simulink model "depth_follower"  (R2019a)
settings: Solver=FixedStepAuto  StartTime=0.0  StopTime=inf  FixedStep=0.1  RelTol=1e-3
model workspace (MAT data in the model file):
  SL_ROS_VariableLengthArrays_MaxSizes.CommonInfo.ArrayTruncateAction = 'EmitWarning'
  SL_ROS_VariableLengthArrays_MaxSizes.MsgTypeMap = containers.Map
  SL_ROS_VariableLengthArrays_MaxSizes.MsgTypeMap.serialization.keys = {'sensor_msgs/Image'}
  SL_ROS_VariableLengthArrays_MaxSizes.MsgTypeMap.serialization.values{1}(1).PropertyName = 'Data'
  SL_ROS_VariableLengthArrays_MaxSizes.MsgTypeMap.serialization.values{1}(1).DataType = 'uint8'
  SL_ROS_VariableLengthArrays_MaxSizes.MsgTypeMap.serialization.values{1}(1).MaxLength = 614400
  SL_ROS_VariableLengthArrays_MaxSizes.MsgTypeMap.serialization.values{1}(2).PropertyName = 'Encoding'
  SL_ROS_VariableLengthArrays_MaxSizes.MsgTypeMap.serialization.values{1}(2).DataType = 'uint8'
  SL_ROS_VariableLengthArrays_MaxSizes.MsgTypeMap.serialization.values{1}(2).MaxLength = 128
  SL_ROS_VariableLengthArrays_MaxSizes.MsgTypeMap.serialization.uniformity = 0
  SL_ROS_VariableLengthArrays_MaxSizes.MsgTypeMap.serialization.keyType = 'char'
  SL_ROS_VariableLengthArrays_MaxSizes.MsgTypeMap.serialization.valueType = 'any'
undefined symbols (not defined in the file): Angular, Linear
libraries: robotlib x5, visionsinks x1
settings Model: EnablePacing=on  Creator=scastro  LastModifiedBy=scastro
settings OptimizationCC: EnhancedBackFolding=on  PassReuseOutputArgsAs=Individual arguments  MaxStackSize=64  OptimizeBlockOrder=speed  DifferentSizesBufferReuse=on  OptimizationCustomize=off
settings DebuggingCC: ParameterTunabilityLossMsg=error
settings HardwareCC: ProdBitPerPointer=32  ProdBitPerSizeT=32  ProdBitPerPtrDiffT=32  ProdLargestAtomicFloat=None  ProdIntDivRoundTo=Undefined  ProdEndianess=Unspecified  ProdWordSize=32  ProdHWDeviceType=Generic->Unspecified (assume 32-bit Generic)
settings RTWCC: SystemTargetFile=ert.tlc  HardwareBoard=Robot Operating System (ROS)  TLCOptions="-aInlineSetEventsForThisBaseRateFcn=TLC_FALSE -aSuppressMultiTaskScheduler=TLC_FALSE  -aRateBasedStepFcn=0"  TemplateMakefile=ert_default_tmf  GenerateReport=on  Toolchain=Catkin  IncludeHyperlinkInReport=on  LaunchReport=on  TargetLang=C++  GenerateTraceInfo=on  GenerateTraceReport=on  GenerateTraceReportSl=on  GenerateTraceReportSf=on  GenerateTraceReportEml=on
settings CodeAppCC: ForceParamTrailComments=on  IgnoreCustomStorageClasses=off  OperatorAnnotations=on  SimulinkDataObjDesc=on  SFDataObjDesc=on  InsertBlockDesc=on
settings ERTTargetCC: SupportVariableSizeSignals=on

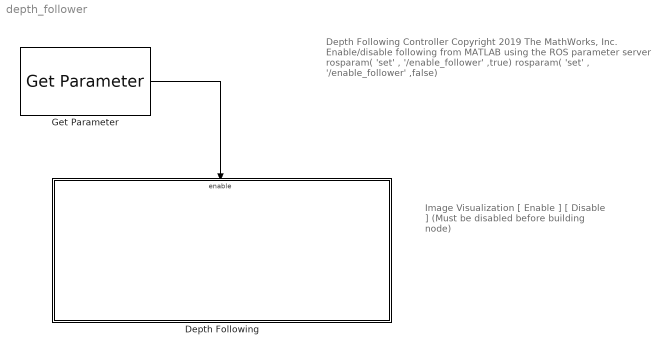
== system depth_follower ==
  note: Depth Following Controller
      | Copyright 2019 The MathWorks, Inc.
      |
      | Enable/disable following from MATLAB
      | using the ROS parameter server
      |
      | rosparam( 'set' , '/enable_follower' ,true)
      | rosparam( 'set' , '/enable_follower' ,false)
  note: Image Visualization
      | [ Enable ] [ Disable ]
      |
      | (Must be disabled before building node)
  Depth Following : Subsystem
  Get Parameter : robotlib/Get Parameter  ParameterSource=Select from ROS network  ParameterName=/enable_follower  ParameterType=boolean  ParameterMaxArrayLength=16  ParameterInitialValue=true  SampleTime=-1  ShowErrorCodeOutput=off  ModelName=depth_follower  BlockId=ParamGet_depth_follower_56
      settings: SourceProductName=Robotics System Toolbox  SourceProductBaseCode=RO
  wires:
  Get Parameter/1 -> Depth Following/Enable

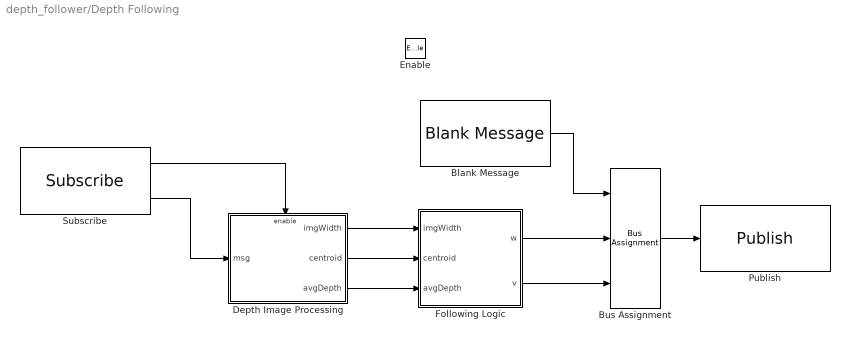
== system depth_follower/Depth Following ==
  Enable : EnablePort
  Blank Message : robotlib/Blank Message  messageClass=Message  entityType=geometry_msgs/Twist  messageType=geometry_msgs/Twist  SampleTime=inf
      settings: SourceProductBaseCode=RO
  Bus Assignment : BusAssignment  AssignedSignals=Angular.Z,Linear.X
  Depth Image Processing : Subsystem
  Following Logic : Subsystem
  Publish : robotlib/Publish  topicSource=Select from ROS network  topic=/mobile_base/commands/velocity  messageType=geometry_msgs/Twist  messageQueueLength=1
      settings: SourceProductBaseCode=RO
  Subscribe : robotlib/Subscribe  topicSource=Select from ROS network  topic=/camera/depth_registered/image_raw  messageType=sensor_msgs/Image  sampleTime=-1  messageQueueLength=1
      settings: SourceProductBaseCode=RO
  wires:
  Blank Message/1 -> Bus Assignment/1
  Depth Image Processing/2(centroid) -> Following Logic/2(centroid)
  Following Logic/1(w) -> Bus Assignment/2
  Following Logic/2(v) -> Bus Assignment/3
  Bus Assignment/1 -> Publish/1
  Depth Image Processing/3(avgDepth) -> Following Logic/3(avgDepth)
  Subscribe/1 -> Depth Image Processing/Enable
  Subscribe/2 -> Depth Image Processing/1(msg)
  Depth Image Processing/1(imgWidth) -> Following Logic/1(imgWidth)

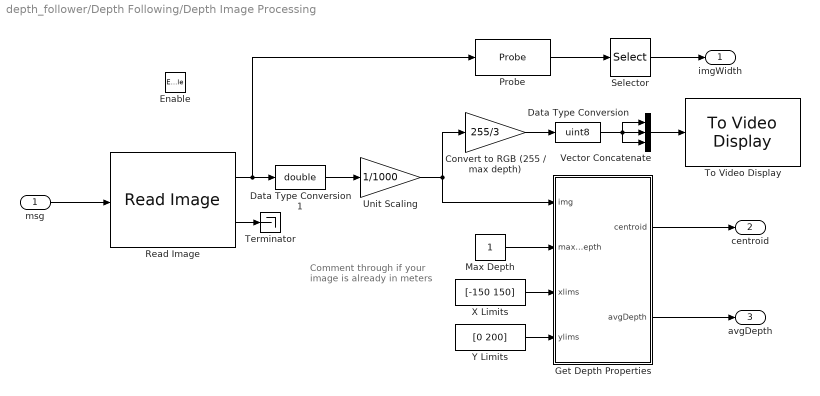
== system depth_follower/Depth Following/Depth Image Processing ==
  note: Comment through if your image is already in meters
  msg : Inport
  Enable : EnablePort
  Convert to RGB (255 / max depth) : Gain  Gain=255/3
  Data Type Conversion : DataTypeConversion  OutDataTypeStr=uint8
  Data Type Conversion1 : DataTypeConversion  OutDataTypeStr=double
  Get Depth Properties : MATLAB Function  TreatAsAtomicUnit=on
  Max Depth : Constant
  Probe : Probe  ProbeWidth=off  ProbeSampleTime=off  ProbeComplexSignal=off  ProbeSignalDimensions=on
  Read Image : robotlib/Read Image  MaximumImageSize=[480, 640]  ImageEncoding=16uc1  ShowAlphaOutput=off  ShowErrorCodeOutput=on  VariableSizeOutputs=off
      settings: SourceProductName=Robotics System Toolbox  SourceProductBaseCode=RO
  Selector : Selector  InputPortWidth=2  IndexOptions=Index vector (dialog)  Indices=2  OutputSizes=1
  Terminator : Terminator
  To Video Display : visionsinks/To Video Display  windowSizeMode=Normal  openAtMdlStart=on  fullScreen=off  videoWindowX=2400  videoWindowY=29  saveWindowSize=off  videoWindowWidth=2400  videoWindowHeight=1471  inputColorFormat=RGB  inputType=Obsolete  imagePorts=One multidimensional signal  OutputDevice=On-screen video monitor  dataOrg=Column-major  isWindowOpen=off
      settings: SourceProductName=Computer Vision Toolbox
  Unit Scaling : Gain  Gain=1/1000
  Vector Concatenate : Concatenate  NumInputs=3  Mode=Multidimensional array  ConcatenateDimension=3
  X Limits : Constant  Value=[-150 150]
  Y Limits : Constant  Value=[0 200]
  imgWidth : Outport
  centroid : Outport  Port=2
  avgDepth : Outport  Port=3
  wires:
  Read Image/1 -> Probe/1, Data Type Conversion1/1
  msg/1 -> Read Image/1
  Read Image/2 -> Terminator/1
  Get Depth Properties/1(centroid) -> centroid/1
  Vector Concatenate/1 -> To Video Display/1
  Convert to RGB (255 / max depth)/1 -> Data Type Conversion/1
  Data Type Conversion/1 -> Vector Concatenate/1, Vector Concatenate/3, Vector Concatenate/2
  Unit Scaling/1 -> Get Depth Properties/1(img), Convert to RGB (255 / max depth)/1
  Data Type Conversion1/1 -> Unit Scaling/1
  Get Depth Properties/2(avgDepth) -> avgDepth/1
  Probe/1 -> Selector/1
  Selector/1 -> imgWidth/1
  Max Depth/1 -> Get Depth Properties/2(maxDepth)
  X Limits/1 -> Get Depth Properties/3(xlims)
  Y Limits/1 -> Get Depth Properties/4(ylims)

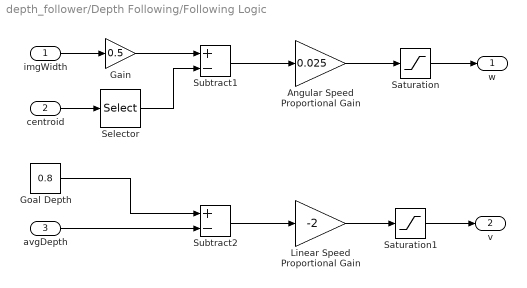
== system depth_follower/Depth Following/Following Logic ==
  imgWidth : Inport
  centroid : Inport  Port=2
  avgDepth : Inport  Port=3
  Angular Speed Proportional Gain : Gain  Gain=0.025
  Gain : Gain  Gain=0.5
  Goal Depth : Constant  Value=0.8
  Linear Speed Proportional Gain : Gain  Gain=-2
  Saturation : Saturate  UpperLimit=1  LowerLimit=-1
  Saturation1 : Saturate  UpperLimit=0.25  LowerLimit=-0.25
  Selector : Selector  InputPortWidth=2  IndexOptions=Index vector (dialog)  Indices=2  OutputSizes=1
  Subtract1 : Sum  Inputs=+-
  Subtract2 : Sum  Inputs=+-
  w : Outport
  v : Outport  Port=2
  wires:
  imgWidth/1 -> Gain/1
  centroid/1 -> Selector/1
  Gain/1 -> Subtract1/1
  Subtract1/1 -> Angular Speed Proportional Gain/1
  Angular Speed Proportional Gain/1 -> Saturation/1
  Saturation/1 -> w/1
  avgDepth/1 -> Subtract2/2
  Goal Depth/1 -> Subtract2/1
  Subtract2/1 -> Linear Speed Proportional Gain/1
  Linear Speed Proportional Gain/1 -> Saturation1/1
  Saturation1/1 -> v/1
  Selector/1 -> Subtract1/2

== matlab function depth_follower/Depth Following/Depth Image Processing/Get Depth Properties ==
  data: img input; centroid output; avgDepth output; maxDepth input; xlims input; ylims input
function [centroid,avgDepth] = getDepthProps(img,maxDepth,xlims,ylims)

% Filter the image
imgSize = size(img);
xIdx = (xlims(1):xlims(2))+imgSize(2)/2;
yIdx = (ylims(1):ylims(2))+imgSize(1)/2;
imgSub = img(yIdx,xIdx);

% Find valid indices based on nonzero and max depth
validIdx = imgSub > 0 & imgSub <= maxDepth;
[r,c] = find(validIdx);

% Compute centroid and average depth
centroid = [mean(r)+yIdx(1);mean(c)+xIdx(1)];
avgDepth = mean(imgSub(validIdx));
